simulink model "sampleModel1790"  (R2023a)
settings: Solver=VariableStepAuto  StartTime=0.0  StopTime=10.0  RelTol=1e-3
libraries: hdlsllib x11
settings Model: Creator=user1  LastModifiedBy=user1

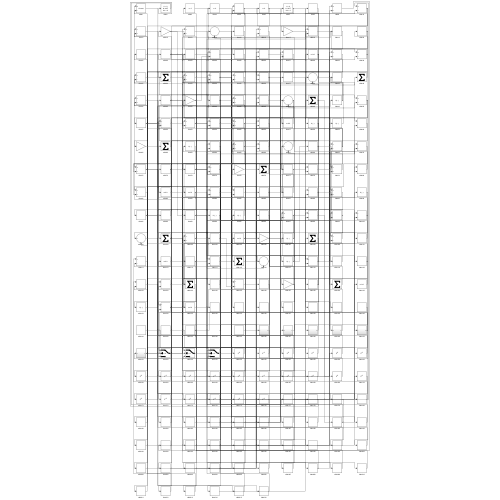
[thumbnail: Simulink's stored preview of the top-level diagram]
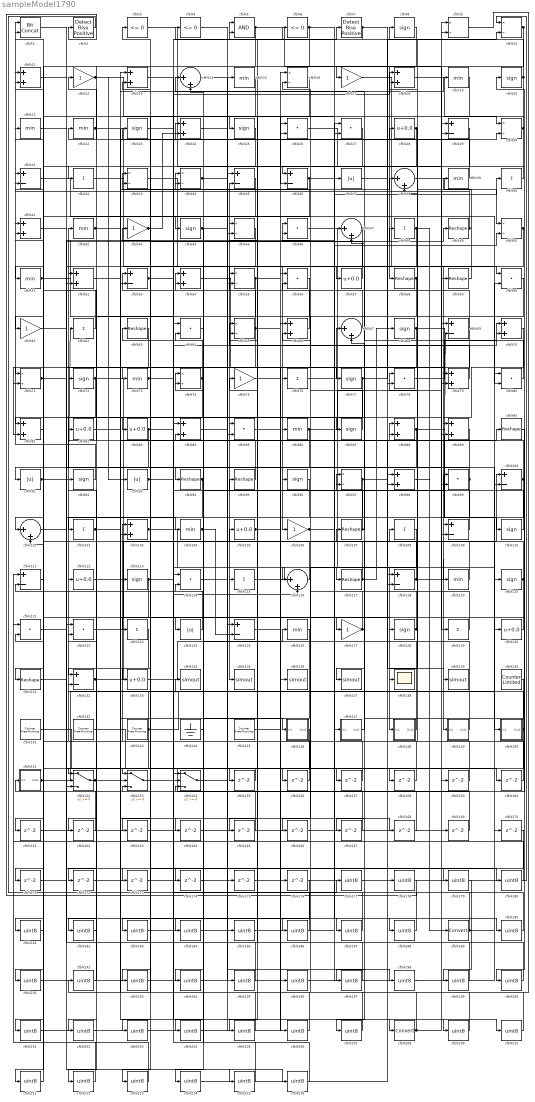
== system sampleModel1790 ==
  cfblk1 : hdlsllib/Logic and Bit Operations/Bit Concat  numInputs=2
  cfblk{9..10,16,30,33..34,45,50,55,65,71,74,97} (13 alike) : Product  Inputs=*/  RndMeth=Zero  SaturateOnIntegerOverflow=on
  cfblk{29,31,35..36,53,69,100,109,111,118,125,132} (12 alike) : Sum  Inputs=+-
  cfblk{14,38,47,67,101,116} (6 alike) : Sum  Inputs=|++
  cfblk{32,40,48,62,76,102,108,115,123,129} (10 alike) : Sum  Inputs=+
  cfblk{11,13,18,24,41,52,54,66,70,79,81,84,88..89,98,103} (16 alike) : Sum
  cfblk{15,19,21..22,39,42,51,73,86,104,119,126} (12 alike) : MinMax
  cfblk{28,57,82..83,105,112,130,133} (8 alike) : Bias  Bias=0.0  SaturateOnIntegerOverflow=off
  cfblk{12,17,43,61,75,106,127} (7 alike) : Gain
  cfblk{49,58..59,63,90,94..95,107,117,131} (10 alike) : Reshape
  cfblk{8,20,23,25,44,68,72,77,87,92,96,110,113,120,128} (15 alike) : Signum
  cfblk{26..27,46,56,60,64,78,80,85,99,114,121..122} (13 alike) : DotProduct  OutDataTypeStr=Inherit: Inherit via internal rule
  cfblk{37,91,93,124} (4 alike) : Abs  SaturateOnIntegerOverflow=off
  cfblk{134..137,139} (5 alike) : ToWorkspace  VariableName=simout  SaveFormat=Timeseries  SampleTime=-1
  cfblk138 : Scope
  cfblk140 : hdlsllib/Sources/Counter Limited  uplimit=7  tsamp=-1
  cfblk{141..143,145} (4 alike) : hdlsllib/Sources/Counter Free-Running  NumBits=16  tsamp=-1
  cfblk144 : Ground
  cfblk146 : Subsystem
      settings: LibrarySourceBlock=|
      | hdlsllib/Ports &
      | Subsystems/Subsystem
  cfblk147 : Subsystem
      settings: LibrarySourceBlock=|
      | hdlsllib/Ports &
      | Subsystems/Subsystem
  cfblk148 : Subsystem
      settings: LibrarySourceBlock=|
      | hdlsllib/Ports &
      | Subsystems/Subsystem
  cfblk149 : Subsystem
      settings: LibrarySourceBlock=|
      | hdlsllib/Ports &
      | Subsystems/Subsystem
  cfblk150 : Subsystem
      settings: LibrarySourceBlock=|
      | hdlsllib/Ports &
      | Subsystems/Subsystem
  cfblk151 : Subsystem
      settings: LibrarySourceBlock=|
      | hdlsllib/Ports &
      | Subsystems/Subsystem
  cfblk152 : Switch  SaturateOnIntegerOverflow=off  InputSameDT=off
  cfblk153 : Switch  SaturateOnIntegerOverflow=off  InputSameDT=off
  cfblk154 : Switch  SaturateOnIntegerOverflow=off  InputSameDT=off
  cfblk{155..176} (22 alike) : Delay  SampleTime=1
  cfblk{177..188,190..207,209..216} (38 alike) : DataTypeConversion  OutDataTypeStr=uint8  SaturateOnIntegerOverflow=off  RndMeth=Floor
  cfblk189 : DataTypeConversion  SaturateOnIntegerOverflow=off  RndMeth=Floor
  cfblk2 : hdlsllib/Logic and Bit Operations/Detect Rise Positive  vinit=0  OutDataTypeStr=boolean
  cfblk208 : DataTypeConversion  SaturateOnIntegerOverflow=off  RndMeth=Floor
  cfblk3 : hdlsllib/Logic and Bit Operations/Compare To Zero  relop=<=  OutDataTypeStr=boolean
  cfblk4 : hdlsllib/Logic and Bit Operations/Compare To Zero  relop=<=  OutDataTypeStr=boolean
  cfblk5 : Logic  AllPortsSameDT=off  OutDataTypeStr=boolean
  cfblk6 : hdlsllib/Logic and Bit Operations/Compare To Zero  relop=<=  OutDataTypeStr=boolean
  cfblk7 : hdlsllib/Logic and Bit Operations/Detect Rise Positive  vinit=0  OutDataTypeStr=boolean
  wires:
  cfblk67/1 -> cfblk53/1
  cfblk95/1 -> cfblk42/1
  cfblk10/1 -> cfblk58/1, cfblk85/2
  cfblk115/1 -> cfblk117/1
  cfblk72/1 -> cfblk124/1, cfblk181/1
  cfblk92/1 -> cfblk1/1
  cfblk49/1 -> cfblk31/1, cfblk4/1
  cfblk22/1 -> cfblk135/1, cfblk30/2, cfblk44/1
  cfblk91/1 -> cfblk62/1, cfblk173/1
  cfblk140/1 -> cfblk103/1
  cfblk36/1 -> cfblk89/2, cfblk161/1
  cfblk17/1 -> cfblk60/1
  cfblk94/1 -> cfblk162/1, cfblk163/1
  cfblk125/1 -> cfblk16/1
  cfblk120/1 -> cfblk21/1, cfblk171/1
  cfblk110/1 -> cfblk54/1
  cfblk141/1 -> cfblk20/1
  cfblk40/1 -> cfblk36/1
  cfblk132/1 -> cfblk100/1, cfblk146/1(In1)
  cfblk32/1 -> cfblk106/1
  cfblk33/1 -> cfblk149/1(In1)
  cfblk150/1(Out1) -> cfblk72/1, cfblk134/1, cfblk194/1
  cfblk129/1 -> cfblk22/1
  cfblk51/1 -> cfblk114/1, cfblk40/1, cfblk190/1
  cfblk50/1 -> cfblk82/1, cfblk152/1
  cfblk68/1 -> cfblk110/1, cfblk184/1
  cfblk16/1 -> cfblk36/2
  cfblk8/1 -> cfblk17/1
  cfblk46/1 -> cfblk148/1(In1)
  cfblk99/1 -> cfblk96/1, cfblk193/1
  cfblk113/1 -> cfblk97/1, cfblk123/1
  cfblk69/1 -> cfblk23/1, cfblk47/2, cfblk18/1, cfblk71/2
  cfblk38/1 -> cfblk50/1
  cfblk5/1 -> cfblk71/1, cfblk109/2
  cfblk71/1 -> cfblk94/1, cfblk216/1
  cfblk78/1 -> cfblk70/1
  cfblk124/1 -> cfblk41/1
  cfblk53/1 -> cfblk7/1, cfblk78/2
  cfblk61/1 -> cfblk48/1
  cfblk149/1(Out1) -> cfblk34/1
  cfblk19/1 -> cfblk73/1
  cfblk118/1 -> cfblk69/2, cfblk24/1
  cfblk98/1 -> cfblk189/1
  cfblk102/1 -> cfblk157/1, cfblk210/1
  cfblk76/1 -> cfblk67/1
  cfblk107/1 -> cfblk67/2, cfblk74/2
  cfblk58/1 -> cfblk132/1, cfblk76/1
  cfblk122/1 -> cfblk108/1
  cfblk77/1 -> cfblk81/1, cfblk10/2
  cfblk34/1 -> cfblk87/1, cfblk160/1
  cfblk127/1 -> cfblk95/1, cfblk167/1
  cfblk55/1 -> cfblk83/1, cfblk57/1
  cfblk35/1 -> cfblk103/2
  cfblk20/1 -> cfblk85/1, cfblk45/2, cfblk6/1
  cfblk153/1 -> cfblk49/1
  cfblk88/1 -> cfblk120/1, cfblk197/1
  cfblk39/1 -> cfblk12/1
  cfblk63/1 -> cfblk81/2
  cfblk28/1 -> cfblk138/1, cfblk202/1
  cfblk37/1 -> cfblk118/1
  cfblk66/1 -> cfblk35/2
  cfblk26/1 -> cfblk129/1
  cfblk131/1 -> cfblk46/1
  cfblk44/1 -> cfblk118/2, cfblk204/1
  cfblk147/1(Out1) -> cfblk107/1
  cfblk148/1(Out1) -> cfblk66/2
  cfblk25/1 -> cfblk61/1
  cfblk109/1 -> cfblk54/2
  cfblk89/1 -> cfblk137/1
  cfblk82/1 -> cfblk128/1
  cfblk116/1 -> cfblk5/1
  cfblk48/1 -> cfblk169/1, cfblk207/1
  cfblk130/1 -> cfblk127/1
  cfblk45/1 -> cfblk53/2
  cfblk83/1 -> cfblk131/1, cfblk116/1
  cfblk11/1 -> cfblk77/1
  cfblk1/1 -> cfblk79/1
  cfblk87/1 -> cfblk16/2
  cfblk3/1 -> cfblk119/1
  cfblk41/1 -> cfblk86/1
  cfblk13/1 -> cfblk208/1
  cfblk133/1 -> cfblk126/1
  cfblk97/1 -> cfblk115/1, cfblk90/1
  cfblk59/1 -> cfblk39/1
  cfblk103/1 -> cfblk150/1(In1), cfblk43/1
  cfblk80/1 -> cfblk14/1
  cfblk52/1 -> cfblk38/1
  cfblk31/1 -> cfblk80/2
  cfblk6/1 -> cfblk32/1, cfblk188/1
  cfblk70/1 -> cfblk89/1
  cfblk43/1 -> cfblk133/1, cfblk24/2
  cfblk106/1 -> cfblk50/2, cfblk180/1
  cfblk104/1 -> cfblk74/1, cfblk125/2
  cfblk7/1 -> cfblk5/2, cfblk139/1
  cfblk4/1 -> cfblk125/1
  cfblk57/1 -> cfblk3/1
  cfblk12/1 -> cfblk47/1, cfblk93/1
  cfblk62/1 -> cfblk11/1
  cfblk119/1 -> cfblk78/1
  cfblk152/1 -> cfblk113/1, cfblk88/1
  cfblk117/1 -> cfblk45/1, cfblk68/1
  cfblk60/1 -> cfblk102/1
  cfblk105/1 -> cfblk99/1, cfblk88/2
  cfblk74/1 -> cfblk101/1, cfblk33/1
  cfblk30/1 -> cfblk25/1, cfblk51/1
  cfblk65/1 -> cfblk153/2, cfblk14/2, cfblk28/1
  cfblk18/1 -> cfblk30/1
  cfblk81/1 -> cfblk101/2
  cfblk54/1 -> cfblk136/1
  cfblk143/1 -> cfblk92/1, cfblk59/1, cfblk191/1, cfblk213/1
  cfblk73/1 -> cfblk70/2, cfblk18/2, cfblk168/1
  cfblk21/1 -> cfblk104/1
  cfblk128/1 -> cfblk8/1, cfblk33/2
  cfblk86/1 -> cfblk29/1, cfblk152/3
  cfblk29/1 -> cfblk91/1
  cfblk112/1 -> cfblk19/1
  cfblk42/1 -> cfblk99/2, cfblk164/1
  cfblk93/1 -> cfblk97/2, cfblk116/2
  cfblk100/1 -> cfblk109/1, cfblk52/1
  cfblk47/1 -> cfblk55/1, cfblk152/2
  cfblk144/1 -> cfblk34/2
  cfblk151/1(Out1) -> cfblk100/2, cfblk215/1
  cfblk79/1 -> cfblk65/1
  cfblk23/1 -> cfblk155/1
  cfblk155/1 -> cfblk153/1
  cfblk101/1 -> cfblk156/1
  cfblk156/1 -> cfblk31/2
  cfblk157/1 -> cfblk41/2
  cfblk114/1 -> cfblk158/1
  cfblk158/1 -> cfblk132/2
  cfblk159/1 -> cfblk38/2
  cfblk160/1 -> cfblk66/1
  cfblk161/1 -> cfblk35/1
  cfblk162/1 -> cfblk1/2
  cfblk163/1 -> cfblk29/2
  cfblk96/1 -> cfblk165/1
  cfblk165/1 -> cfblk11/2
  cfblk108/1 -> cfblk166/1
  cfblk166/1 -> cfblk69/1
  cfblk167/1 -> cfblk46/2
  cfblk168/1 -> cfblk153/3
  cfblk169/1 -> cfblk65/2
  cfblk171/1 -> cfblk52/2
  cfblk123/1 -> cfblk172/1
  cfblk172/1 -> cfblk10/1
  cfblk173/1 -> cfblk55/2
  cfblk126/1 -> cfblk174/1
  cfblk174/1 -> cfblk79/2
  cfblk24/1 -> cfblk175/1
  cfblk175/1 -> cfblk80/1
  cfblk2/1 -> cfblk177/1
  cfblk177/1 -> cfblk130/1
  cfblk178/1 -> cfblk2/1
  cfblk121/1 -> cfblk179/1
  cfblk180/1 -> cfblk121/1
  cfblk181/1 -> cfblk121/2
  cfblk27/1 -> cfblk182/1
  cfblk182/1 -> cfblk112/1
  cfblk170/1 -> cfblk183/1
  cfblk183/1 -> cfblk27/1
  cfblk184/1 -> cfblk27/2
  cfblk154/1 -> cfblk185/1
  cfblk185/1 -> cfblk37/1
  cfblk14/1 -> cfblk186/1
  cfblk186/1 -> cfblk154/1
  cfblk164/1 -> cfblk187/1
  cfblk187/1 -> cfblk154/2
  cfblk188/1 -> cfblk154/3
  cfblk189/1 -> cfblk170/1, cfblk105/1
  cfblk190/1 -> cfblk98/1
  cfblk191/1 -> cfblk98/2
  cfblk9/1 -> cfblk192/1
  cfblk192/1 -> cfblk122/2
  cfblk193/1 -> cfblk9/1
  cfblk194/1 -> cfblk9/2
  cfblk142/1 -> cfblk195/1
  cfblk195/1 -> cfblk122/1
  cfblk75/1 -> cfblk196/1
  cfblk196/1 -> cfblk147/1(In1)
  cfblk197/1 -> cfblk75/1
  cfblk84/1 -> cfblk198/1
  cfblk198/1 -> cfblk60/2
  cfblk179/1 -> cfblk199/1
  cfblk199/1 -> cfblk84/1
  cfblk90/1 -> cfblk200/1
  cfblk200/1 -> cfblk84/2
  cfblk15/1 -> cfblk201/1
  cfblk201/1 -> cfblk26/1
  cfblk202/1 -> cfblk15/1
  cfblk176/1 -> cfblk203/1
  cfblk203/1 -> cfblk26/2
  cfblk204/1 -> cfblk176/1
  cfblk56/1 -> cfblk205/1
  cfblk205/1 -> cfblk63/1
  cfblk145/1 -> cfblk206/1
  cfblk206/1 -> cfblk56/1
  cfblk207/1 -> cfblk56/2
  cfblk208/1 -> cfblk159/1, cfblk114/2
  cfblk85/1 -> cfblk209/1
  cfblk209/1 -> cfblk13/1
  cfblk210/1 -> cfblk13/2
  cfblk111/1 -> cfblk211/1
  cfblk211/1 -> cfblk151/1(In1)
  cfblk146/1(Out1) -> cfblk212/1
  cfblk212/1 -> cfblk111/1
  cfblk213/1 -> cfblk111/2
  cfblk64/1 -> cfblk214/1
  cfblk214/1 -> cfblk178/1
  cfblk215/1 -> cfblk64/1
  cfblk216/1 -> cfblk64/2

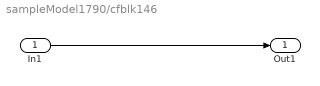
== system sampleModel1790/cfblk146 ==
  In1 : Inport
  Out1 : Outport
  wires:
  In1/1 -> Out1/1

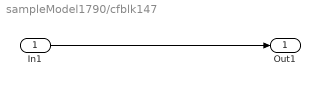
== system sampleModel1790/cfblk147 ==
  In1 : Inport
  Out1 : Outport
  wires:
  In1/1 -> Out1/1

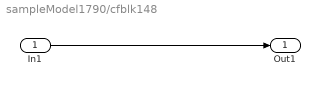
== system sampleModel1790/cfblk148 ==
  In1 : Inport
  Out1 : Outport
  wires:
  In1/1 -> Out1/1

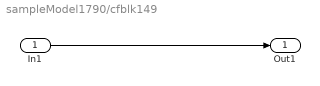
== system sampleModel1790/cfblk149 ==
  In1 : Inport
  Out1 : Outport
  wires:
  In1/1 -> Out1/1

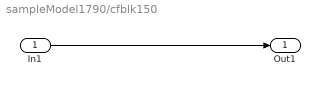
== system sampleModel1790/cfblk150 ==
  In1 : Inport
  Out1 : Outport
  wires:
  In1/1 -> Out1/1

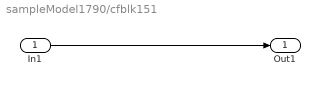
== system sampleModel1790/cfblk151 ==
  In1 : Inport
  Out1 : Outport
  wires:
  In1/1 -> Out1/1
